simulink model "self_balance_pid_discr_torquereverse_pidzn2_nonlinear"  (R2023b)
settings: Solver=FixedStepAuto  StartTime=0.0  StopTime=10  FixedStep=0.001  RelTol=1e-3
settings Model: Creator=emamaker  LastModifiedBy=emamaker

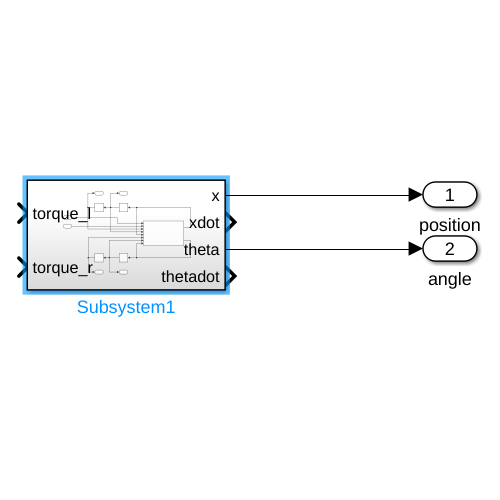
[thumbnail: Simulink's stored preview of the top-level diagram]
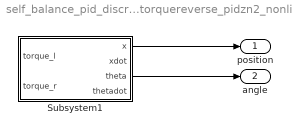
== system self_balance_pid_discr_torquereverse_pidzn2_nonlinear ==
  Subsystem1 : Subsystem
  position : Outport
  angle : Outport  Port=2
  wires:
  Subsystem1/1(x) -> position/1
  Subsystem1/3(theta) -> angle/1

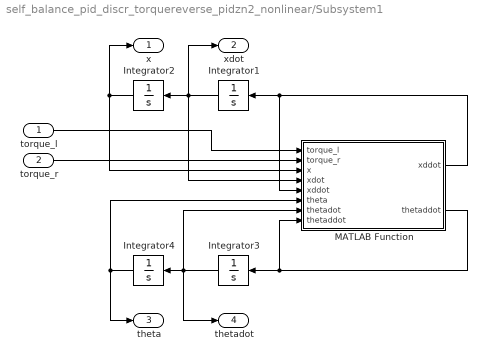
== system self_balance_pid_discr_torquereverse_pidzn2_nonlinear/Subsystem1 ==
  torque_l : Inport
  torque_r : Inport  Port=2
  Integrator{1..4} (4 alike) : Integrator
  MATLAB Function : MATLAB Function  TreatAsAtomicUnit=on
  x : Outport
  xdot : Outport  Port=2
  theta : Outport  Port=3
  thetadot : Outport  Port=4
  wires:
  MATLAB Function/1(xddot) -> Integrator1/1, MATLAB Function/5("xddot ")
  MATLAB Function/2(thetaddot) -> Integrator3/1, MATLAB Function/8("thetaddot ")
  Integrator3/1 -> thetadot/1, Integrator4/1, MATLAB Function/7(thetadot)
  Integrator1/1 -> Integrator2/1, MATLAB Function/4(xdot), xdot/1
  Integrator4/1 -> theta/1, MATLAB Function/6(theta)
  Integrator2/1 -> x/1, MATLAB Function/3(x)
  torque_r/1 -> MATLAB Function/2(torque_r)
  torque_l/1 -> MATLAB Function/1(torque_l)

== matlab function self_balance_pid_discr_torquereverse_pidzn2_nonlinear/Subsystem1/MATLAB Function ==
  data: torque_l input; torque_r input; x input; xdot input; xddot input; theta input; xddot output; thetadot input; thetaddot output; thetaddot input
function [xddot, thetaddot]= fcn(torque_l, torque_r, x, xdot, xddot, theta, thetadot, thetaddot)


b = 0.1;
g = 9.81;
M_wheel = 0.012;
M_body=0.232;

r = 0.032;
l = 0.035;

% inertia
I_wheel = (M_wheel*r^2); %placeholder
I_body = M_body*l^2/3; %placeholder


xddot_num = (torque_l + torque_r) / r - 2*b*xdot/(r^2) + M_body*l*(sin(theta)* thetadot^2 - cos(theta)*thetaddot);
xddot_den = M_body + 2*I_wheel/(r^2) +2*M_wheel;

thetaddot_num = -(torque_l + torque_r) + M_body*l(g*sin(theta) - xddot*cos(theta));
thetaddot_den = I_body + M_body*l^2;


xddot = xddot_num / xddot_den;
thetaddot = thetaddot_num / thetaddot_den;
